simulink model "KF"  (R2023a)
settings: Solver=VariableStepAuto  StartTime=0.0  StopTime=20  RelTol=1e-3
settings Model: Creator=belov  LastModifiedBy=belov

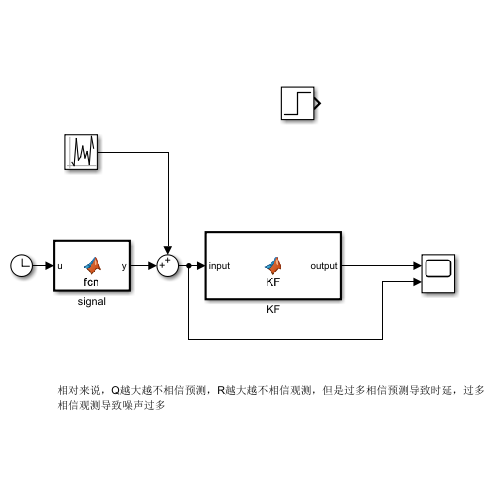
[thumbnail: Simulink's stored preview of the top-level diagram]
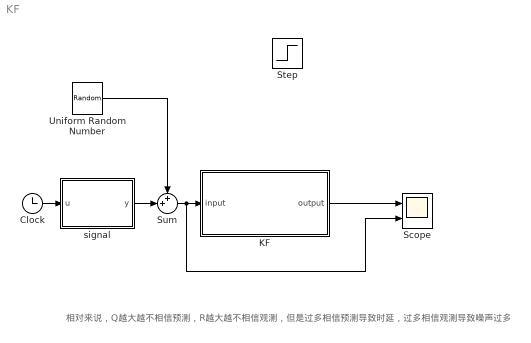
== system KF ==
  note: 相对来说，Q越大越不相信预测，R越大越不相信观测，但是过多相信预测导致时延，过多相信观测导致噪声过多
  Clock : Clock
  KF : MATLAB Function  TreatAsAtomicUnit=on
  Scope : Scope  NumInputPorts=2
  Step : Step  SampleTime=0
  Sum : Sum  Inputs=++|
  Uniform Random Number : UniformRandomNumber  Minimum=-0.05  Maximum=0.05  SampleTime=0.1
  signal : MATLAB Function  TreatAsAtomicUnit=on
  wires:
  Clock/1 -> signal/1(u)
  KF/1(output) -> Scope/1
  signal/1(y) -> Sum/2
  Sum/1 -> Scope/2, KF/1(input)
  Uniform Random Number/1 -> Sum/1

== matlab function KF/KF ==
  data: input input; output output
function output = KF(input)
persistent x_last_last P_last_last;
if(isempty(x_last_last))
    x_last_last = 0;
end
if(isempty(P_last_last))
    P_last_last = 1;
end

F_k = 1;
H_k = 1;

Q_k = 1;
R_k = 4;



x_last_now = F_k * x_last_last;
P_last_now = F_k * P_last_last * F_k' + Q_k;
K_k = P_last_now * H_k' * inv(H_k * P_last_now * H_k' + R_k);
x_now_now = x_last_now + K_k * (input - H_k * x_last_now);
I = eye(size(K_k * H_k));
P_last_last = (I - K_k * H_k) * P_last_now;
x_last_last = x_now_now;

output = x_now_now;

== matlab function KF/signal ==
  data: u input; y output
function y = fcn(u)

y = sin(u);
